simulink model "TV_2017old"  (R2016a)
settings: Solver=FixedStepAuto  StartTime=0.0  StopTime=inf  FixedStep=0.001  RelTol=1e-3
PreLoadFcn:
  | TV_2017_parameters
values from neighbouring files (symbols this model uses):
  battery_voltage = single(530)    [HIL_parameters.m]    (also in HIL_parameters_2018.m; TV_2017_parameters.m; TV_2017_parameters_VD.m)
  car_params = Simulink_Car_params    [HIL_parameters.m]    (also in HIL_parameters_2018.m; TV_2017_parameters.m; TV_2017_parameters_VD.m)
  i_Diff = 16    [HIL_parameters.m]    (also in HIL_parameters_2018.m; TV_2017_parameters.m)
  Kp = 1    [HIL_parameters.m]    (also in HIL_parameters_2018.m; TV_2017_parameters.m; TV_2017_parameters_VD.m)
  motor_data = struct    [HIL_parameters.m]    (also in HIL_parameters_2018.m; TV_2017_parameters.m)
  powerLimitControl = Simulink_el    [HIL_parameters.m]    (also in HIL_parameters_2018.m; TV_2017_parameters.m; TV_2017_parameters_VD.m)
  settings = Simulink_Settings    [HIL_parameters.m]    (also in HIL_parameters_2018.m; TV_2017_parameters.m; TV_2017_parameters_VD.m)
  SpdC_BCC = 0    [HIL_parameters.m]    (also in HIL_parameters_2018.m; TV_2017_parameters.m; TV_2017_parameters_VD.m)
  Speed_Neg_sat = -21    [HIL_parameters.m]    (also in HIL_parameters_2018.m; TV_2017_parameters.m; TV_2017_parameters_VD.m)
  Speed_Pos_sat = 21    [HIL_parameters.m]    (also in HIL_parameters_2018.m; TV_2017_parameters.m; TV_2017_parameters_VD.m)
  SteeringAngleFL = [-23.80 -22.65 -21.50 -20.34 -19.18 -18.03 -16.86 -15.70 -14.53 -13.35 -12.18 -10.99 -9.80 -8.61 -7.40 -6.19 -4.97 -3.75 -2.51 -1.26 0 1.27 2.56 3.85 5.17 6.50 7.84 9.21 10.59 12.00 13.42 14.88 16.36 17.87 19.41 20.99 22.61 24.26 25.97 27.73 29.54]    [CarSetupAnalysis2018.m]    (also in HIL_parameters_2018.m; TV_2017_parameters.m; TV_2017_parameters_VD.m = [-24.129 -22.950 -21.772 -20.593 -19.413 -18.232 -17.050 -15)
  SteeringAngleFR = [-29.54 -27.73 -25.97 -24.26 -22.61 -20.99 -19.41 -17.87 -16.36 -14.88 -13.42 -12.00 -10.59 -9.21 -7.84 -6.50 -5.17 -3.85 -2.56 -1.27 0 1.26 2.51 3.75 4.97 6.19 7.40 8.61 9.80 10.99 12.18 13.35 14.53 15.70 16.86 18.03 19.18 20.34 21.50 22.65 23.80]    [CarSetupAnalysis2018.m]    (also in HIL_parameters_2018.m; TV_2017_parameters.m; TV_2017_parameters_VD.m = [-29.3050 -27.5340 -25.8140 -24.1410 -22.5110 -20.9180 -19.3)
  SteeringWhAngle = [-105 -99.75 -94.5 -89.25 -84 -78.75 -73.5 -68.25 -63 -57.75 -52.5 -47.25 -42 -36.75 -31.5 -26.25 -21.0 -15.75 -10.5 -5.25 0.0 5.25 10.50 15.75 21.00 26.25 31.50 36.75 42.00 47.25 52.50 57.75  63.00 68.25 73.50 78.75 84.00 89.25 94.50 99.75 105.00]    [TV_2017_parameters_VD.m]
  Tn_n = 0    [HIL_parameters.m]    (also in HIL_parameters_2018.m; TV_2017_parameters.m; TV_2017_parameters_VD.m)
  tractionControl = Simulink_tc    [HIL_parameters.m]    (also in HIL_parameters_2018.m; IterativeTractionControlTuning.m; TV_2017_parameters.m; TV_2017_parameters_VD.m)
  yawRateControl = Simulink_yawRate    [HIL_parameters.m]    (also in HIL_parameters_2018.m; TV_2017_parameters.m; TV_2017_parameters_VD.m)
undefined symbols (not defined in the file or in its folder): DiscIntNeverNeededParam, magnitude, speedEstimation, TC_Decr_Gas, TC_Derivative, TC_Incr_Gas, TC_On, TC_Relay_Off, TC_Relay_On
libraries: CarMaker4SL x274, simulink_extras x45, simulink x37, dspfdesign x2
(part 4 of 14)

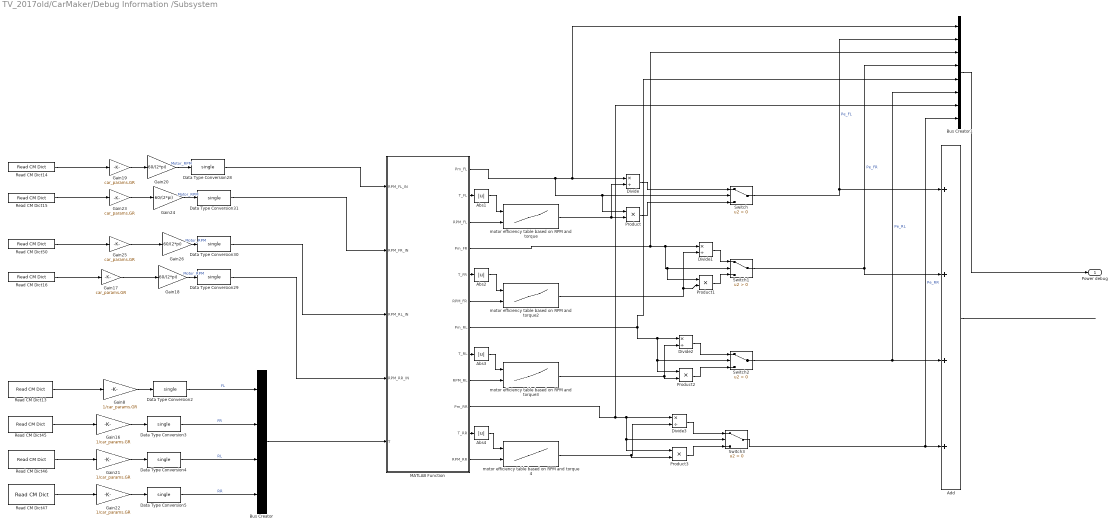
== system TV_2017old/CarMaker/Debug Information /Subsystem ==
  Abs{1..4} (4 alike) : Abs
  Add : Sum  Inputs=++++
  Bus Creator : BusCreator  Inputs=4  OutDataTypeStr=Bus: T_meas
      settings: InheritFromInputs=off
  Bus Creator1 : BusCreator  Inputs=8  OutDataTypeStr=Bus: PowerDebug
      settings: InheritFromInputs=off
  Data Type Conversion{2..5,28..31} (8 alike) : DataTypeConversion  OutDataTypeStr=single
  Divide{,1..3} (4 alike) : Product  Inputs=*/
  Gain{8,16,21..22} (4 alike) : Gain  Gain=1/car_params.GR
  Gain{17,19,23,25} (4 alike) : Gain  Gain=car_params.GR
  Gain{18,20,24,26} (4 alike) : Gain  Gain=60/(2*pi)
  MATLAB Function : MATLAB Function  TreatAsAtomicUnit=on
  Product{,1..3} (4 alike) : Product
  Read CM Dict13 : CarMaker4SL/Read CM Dict  xname=PT.WFL.Trq_Drive  xsync=off
  Read CM Dict14 : CarMaker4SL/Read CM Dict  xname=Car.WheelSpd_FL  xsync=off
  Read CM Dict15 : CarMaker4SL/Read CM Dict  xname=Car.WheelSpd_FR  xsync=off
  Read CM Dict16 : CarMaker4SL/Read CM Dict  xname=Car.WheelSpd_RR  xsync=off
  Read CM Dict45 : CarMaker4SL/Read CM Dict  xname=PT.WFR.Trq_Drive  xsync=off
  Read CM Dict46 : CarMaker4SL/Read CM Dict  xname=PT.WRL.Trq_Drive  xsync=off
  Read CM Dict47 : CarMaker4SL/Read CM Dict  xname=PT.WRR.Trq_Drive  xsync=off
  Read CM Dict50 : CarMaker4SL/Read CM Dict  xname=Car.WheelSpd_RL  xsync=off
  Switch{,1..3} (4 alike) : Switch  Criteria=u2 > Threshold
  motor efficiency table based on RPM and torque : Lookup_n-D  BreakpointsForDimension1=single([1.3,2.7,5.4,7.9,10.4,12.5,14.4,16.0,17.4,18.5,19.6]);  BreakpointsForDimension2=single([500,1000,2000,3000,4000,6000,10000,12000,15000,19000]);  Table=single(reshape([0.6437000036239624,0.5799999833106995,0.44999998807907104,0.3499999940395355,0.28999999165534973,0.23999999463558197,0.20000000298023224,0.17000000178813934,0.14000000059604645,0.12999999523162842,0.10999999940395355,0.7099999785423279,0.699999988079071,0.6100000143051148,0.5099999904632568,0.4399999976158142,0.3799999952316284,0.33000001311302185,0.28999999165534973,0.25,0.2199999988079071,0.20000000298023224,0.7300000190734863,0.7699999809265137,0.7300000190734863,0.6700000166893005,0.6100000143051148,0.550000011920929,0.5,0.44999998807907104,0.4000000059604645,0.36000001430511475,0.33000001311302185,0.7400000095367432,0.800000011920929,0.7900000214576721,0.7400000095367432,0.6899999976158142,0.6399999856948853,0.5899999737739563,0.5400000214576721,0.5,0.46000000834465027,0.41999998688697815,0.75,0.8199999928474426,0.8199999928474426,0.7799999713897705,0.7400000095367432,0.699999988079071,0.6600000262260437,0.6100000143051148,0.5699999928474426,0.5299999713897705,0.49000000953674316,0.7599999904632568,0.8399999737739563,0.8500000238418579,0.8299999833106995,0.800000011920929,0.7699999809265137,0.7400000095367432,0.699999988079071,0.6600000262260437,0.6200000047683716,0.5899999737739563,0.7699999809265137,0.8500000238418579,0.8799999952316284,0.8700000047683716,0.8600000143051148,0.8399999737739563,0.8100000023841858,0.7799999713897705,0.7599999904632568,0.7200000286102295,0.699999988079071,0.7699999809265137,0.8500000238418579,0.8899999856948853,0.8799999952316284,0.8700000047683716,0.8500000238418579,0.8299999833106995,0.8100000023841858,0.7799999713897705,0.7599999904632568,0.7300000190734863,0.7699999809265137,0.8600000143051148,0.8999999761581421,0.8999999761581421,0.8899999856948853,0.8700000047683716,0.8500000238418579,0.8299999833106995,0.8100000023841858,0.7900000214576721,0.6700000166893005,0.7799999713897705,0.8600000143051148,0.8999999761581421,0.9100000262260437,0.8999999761581421,0.8899999856948853,0.8700000047683716,0.8600000143051148,0.8299999833106995,0.7699999809265137,0.699999988079071],11,10));  ExtrapMethod=Clip  UseLastTableValue=on  InternalRulePriority=Speed  RndMeth=Simplest  InputSameDT=on
  motor efficiency table based on RPM and torque 4 : Lookup_n-D  BreakpointsForDimension1=single([1.3,2.7,5.4,7.9,10.4,12.5,14.4,16.0,17.4,18.5,19.6]);  BreakpointsForDimension2=single([500,1000,2000,3000,4000,6000,10000,12000,15000,19000]);  Table=single(reshape([0.6437000036239624,0.5799999833106995,0.44999998807907104,0.3499999940395355,0.28999999165534973,0.23999999463558197,0.20000000298023224,0.17000000178813934,0.14000000059604645,0.12999999523162842,0.10999999940395355,0.7099999785423279,0.699999988079071,0.6100000143051148,0.5099999904632568,0.4399999976158142,0.3799999952316284,0.33000001311302185,0.28999999165534973,0.25,0.2199999988079071,0.20000000298023224,0.7300000190734863,0.7699999809265137,0.7300000190734863,0.6700000166893005,0.6100000143051148,0.550000011920929,0.5,0.44999998807907104,0.4000000059604645,0.36000001430511475,0.33000001311302185,0.7400000095367432,0.800000011920929,0.7900000214576721,0.7400000095367432,0.6899999976158142,0.6399999856948853,0.5899999737739563,0.5400000214576721,0.5,0.46000000834465027,0.41999998688697815,0.75,0.8199999928474426,0.8199999928474426,0.7799999713897705,0.7400000095367432,0.699999988079071,0.6600000262260437,0.6100000143051148,0.5699999928474426,0.5299999713897705,0.49000000953674316,0.7599999904632568,0.8399999737739563,0.8500000238418579,0.8299999833106995,0.800000011920929,0.7699999809265137,0.7400000095367432,0.699999988079071,0.6600000262260437,0.6200000047683716,0.5899999737739563,0.7699999809265137,0.8500000238418579,0.8799999952316284,0.8700000047683716,0.8600000143051148,0.8399999737739563,0.8100000023841858,0.7799999713897705,0.7599999904632568,0.7200000286102295,0.699999988079071,0.7699999809265137,0.8500000238418579,0.8899999856948853,0.8799999952316284,0.8700000047683716,0.8500000238418579,0.8299999833106995,0.8100000023841858,0.7799999713897705,0.7599999904632568,0.7300000190734863,0.7699999809265137,0.8600000143051148,0.8999999761581421,0.8999999761581421,0.8899999856948853,0.8700000047683716,0.8500000238418579,0.8299999833106995,0.8100000023841858,0.7900000214576721,0.6700000166893005,0.7799999713897705,0.8600000143051148,0.8999999761581421,0.9100000262260437,0.8999999761581421,0.8899999856948853,0.8700000047683716,0.8600000143051148,0.8299999833106995,0.7699999809265137,0.699999988079071],11,10));  ExtrapMethod=Clip  UseLastTableValue=on  InternalRulePriority=Speed  RndMeth=Simplest  InputSameDT=on
  motor efficiency table based on RPM and torque2 : Lookup_n-D  BreakpointsForDimension1=single([1.3,2.7,5.4,7.9,10.4,12.5,14.4,16.0,17.4,18.5,19.6]);  BreakpointsForDimension2=single([500,1000,2000,3000,4000,6000,10000,12000,15000,19000]);  Table=single(reshape([0.6437000036239624,0.5799999833106995,0.44999998807907104,0.3499999940395355,0.28999999165534973,0.23999999463558197,0.20000000298023224,0.17000000178813934,0.14000000059604645,0.12999999523162842,0.10999999940395355,0.7099999785423279,0.699999988079071,0.6100000143051148,0.5099999904632568,0.4399999976158142,0.3799999952316284,0.33000001311302185,0.28999999165534973,0.25,0.2199999988079071,0.20000000298023224,0.7300000190734863,0.7699999809265137,0.7300000190734863,0.6700000166893005,0.6100000143051148,0.550000011920929,0.5,0.44999998807907104,0.4000000059604645,0.36000001430511475,0.33000001311302185,0.7400000095367432,0.800000011920929,0.7900000214576721,0.7400000095367432,0.6899999976158142,0.6399999856948853,0.5899999737739563,0.5400000214576721,0.5,0.46000000834465027,0.41999998688697815,0.75,0.8199999928474426,0.8199999928474426,0.7799999713897705,0.7400000095367432,0.699999988079071,0.6600000262260437,0.6100000143051148,0.5699999928474426,0.5299999713897705,0.49000000953674316,0.7599999904632568,0.8399999737739563,0.8500000238418579,0.8299999833106995,0.800000011920929,0.7699999809265137,0.7400000095367432,0.699999988079071,0.6600000262260437,0.6200000047683716,0.5899999737739563,0.7699999809265137,0.8500000238418579,0.8799999952316284,0.8700000047683716,0.8600000143051148,0.8399999737739563,0.8100000023841858,0.7799999713897705,0.7599999904632568,0.7200000286102295,0.699999988079071,0.7699999809265137,0.8500000238418579,0.8899999856948853,0.8799999952316284,0.8700000047683716,0.8500000238418579,0.8299999833106995,0.8100000023841858,0.7799999713897705,0.7599999904632568,0.7300000190734863,0.7699999809265137,0.8600000143051148,0.8999999761581421,0.8999999761581421,0.8899999856948853,0.8700000047683716,0.8500000238418579,0.8299999833106995,0.8100000023841858,0.7900000214576721,0.6700000166893005,0.7799999713897705,0.8600000143051148,0.8999999761581421,0.9100000262260437,0.8999999761581421,0.8899999856948853,0.8700000047683716,0.8600000143051148,0.8299999833106995,0.7699999809265137,0.699999988079071],11,10));  ExtrapMethod=Clip  UseLastTableValue=on  InternalRulePriority=Speed  RndMeth=Simplest  InputSameDT=on
  motor efficiency table based on RPM and torque3 : Lookup_n-D  BreakpointsForDimension1=single([1.3,2.7,5.4,7.9,10.4,12.5,14.4,16.0,17.4,18.5,19.6]);  BreakpointsForDimension2=single([500,1000,2000,3000,4000,6000,10000,12000,15000,19000]);  Table=single(reshape([0.6437000036239624,0.5799999833106995,0.44999998807907104,0.3499999940395355,0.28999999165534973,0.23999999463558197,0.20000000298023224,0.17000000178813934,0.14000000059604645,0.12999999523162842,0.10999999940395355,0.7099999785423279,0.699999988079071,0.6100000143051148,0.5099999904632568,0.4399999976158142,0.3799999952316284,0.33000001311302185,0.28999999165534973,0.25,0.2199999988079071,0.20000000298023224,0.7300000190734863,0.7699999809265137,0.7300000190734863,0.6700000166893005,0.6100000143051148,0.550000011920929,0.5,0.44999998807907104,0.4000000059604645,0.36000001430511475,0.33000001311302185,0.7400000095367432,0.800000011920929,0.7900000214576721,0.7400000095367432,0.6899999976158142,0.6399999856948853,0.5899999737739563,0.5400000214576721,0.5,0.46000000834465027,0.41999998688697815,0.75,0.8199999928474426,0.8199999928474426,0.7799999713897705,0.7400000095367432,0.699999988079071,0.6600000262260437,0.6100000143051148,0.5699999928474426,0.5299999713897705,0.49000000953674316,0.7599999904632568,0.8399999737739563,0.8500000238418579,0.8299999833106995,0.800000011920929,0.7699999809265137,0.7400000095367432,0.699999988079071,0.6600000262260437,0.6200000047683716,0.5899999737739563,0.7699999809265137,0.8500000238418579,0.8799999952316284,0.8700000047683716,0.8600000143051148,0.8399999737739563,0.8100000023841858,0.7799999713897705,0.7599999904632568,0.7200000286102295,0.699999988079071,0.7699999809265137,0.8500000238418579,0.8899999856948853,0.8799999952316284,0.8700000047683716,0.8500000238418579,0.8299999833106995,0.8100000023841858,0.7799999713897705,0.7599999904632568,0.7300000190734863,0.7699999809265137,0.8600000143051148,0.8999999761581421,0.8999999761581421,0.8899999856948853,0.8700000047683716,0.8500000238418579,0.8299999833106995,0.8100000023841858,0.7900000214576721,0.6700000166893005,0.7799999713897705,0.8600000143051148,0.8999999761581421,0.9100000262260437,0.8999999761581421,0.8899999856948853,0.8700000047683716,0.8600000143051148,0.8299999833106995,0.7699999809265137,0.699999988079071],11,10));  ExtrapMethod=Clip  UseLastTableValue=on  InternalRulePriority=Speed  RndMeth=Simplest  InputSameDT=on
  Power debug : Outport
  wires:
  motor efficiency table based on RPM and torque 4/1 -> Product3/2, Divide3/2
  motor efficiency table based on RPM and torque3/1 -> Product2/2, Divide2/2
  Divide1/1 -> Switch1/1
  Product1/1 -> Switch1/3
  MATLAB Function/3(RPM_FL) -> motor efficiency table based on RPM and torque/2
  MATLAB Function/10(Pm_RR) -> Bus Creator1/7, Switch3/2, Product3/1, Divide3/1
  MATLAB Function/2(T_FL) -> Abs1/1
  MATLAB Function/8(T_RL) -> Abs3/1
  Abs4/1 -> motor efficiency table based on RPM and torque 4/1
  Abs2/1 -> motor efficiency table based on RPM and torque2/1
  Data Type Conversion28/1 -> MATLAB Function/1(RPM_FL_IN)
  MATLAB Function/5(T_FR) -> Abs2/1
  MATLAB Function/11(T_RR) -> Abs4/1
  MATLAB Function/12(RPM_RR) -> motor efficiency table based on RPM and torque 4/2
  MATLAB Function/1(Pm_FL) -> Product/1, Switch/2, Divide/1, Bus Creator1/1
  MATLAB Function/7(Pm_RL) -> Switch2/2, Product2/1, Divide2/1, Bus Creator1/5
  Data Type Conversion31/1 -> MATLAB Function/2(RPM_FR_IN)
  Data Type Conversion30/1 -> MATLAB Function/3(RPM_RL_IN)
  Divide/1 -> Switch/1
  Product/1 -> Switch/3
  Data Type Conversion29/1 -> MATLAB Function/4(RPM_RR_IN)
  Bus Creator/1 -> MATLAB Function/5(T)
  motor efficiency table based on RPM and torque/1 -> Divide/2, Product/2
  MATLAB Function/4(Pm_FR) -> Bus Creator1/3, Product1/1, Switch1/2, Divide1/1
  Abs1/1 -> motor efficiency table based on RPM and torque/1
  motor efficiency table based on RPM and torque2/1 -> Divide1/2, Product1/2
  MATLAB Function/6(RPM_FR) -> motor efficiency table based on RPM and torque2/2
  Switch/1 -> Bus Creator1/2, Add/1  "Pe_FL"
  MATLAB Function/9(RPM_RL) -> motor efficiency table based on RPM and torque3/2
  Abs3/1 -> motor efficiency table based on RPM and torque3/1
  Divide2/1 -> Switch2/1
  Divide3/1 -> Switch3/1
  Read CM Dict13/1 -> Gain8/1
  Read CM Dict46/1 -> Gain21/1
  Read CM Dict45/1 -> Gain16/1
  Product3/1 -> Switch3/3
  Switch2/1 -> Bus Creator1/6, Add/3  "Pe_RL"
  Product2/1 -> Switch2/3
  Switch1/1 -> Bus Creator1/4, Add/2  "Pe_FR"
  Switch3/1 -> Add/4, Bus Creator1/8  "Pe_RR"
  Gain24/1 -> Data Type Conversion31/1  "Motor_RPM"
  Read CM Dict15/1 -> Gain23/1
  Gain8/1 -> Data Type Conversion2/1
  Gain22/1 -> Data Type Conversion5/1
  Read CM Dict50/1 -> Gain25/1
  Gain23/1 -> Gain24/1
  Gain19/1 -> Gain20/1
  Bus Creator1/1 -> Power debug/1
  Gain18/1 -> Data Type Conversion29/1  "Motor_RPM"
  Gain26/1 -> Data Type Conversion30/1  "Motor_RPM"
  Read CM Dict14/1 -> Gain19/1
  Data Type Conversion4/1 -> Bus Creator/3  "RL"
  Add/1 -> ?
  Read CM Dict16/1 -> Gain17/1
  Gain17/1 -> Gain18/1
  Data Type Conversion3/1 -> Bus Creator/2  "FR"
  Gain25/1 -> Gain26/1
  Gain16/1 -> Data Type Conversion3/1
  Gain21/1 -> Data Type Conversion4/1
  Data Type Conversion2/1 -> Bus Creator/1  "FL"
  Gain20/1 -> Data Type Conversion28/1  "Motor_RPM"
  Data Type Conversion5/1 -> Bus Creator/4  "RR"
  Read CM Dict47/1 -> Gain22/1

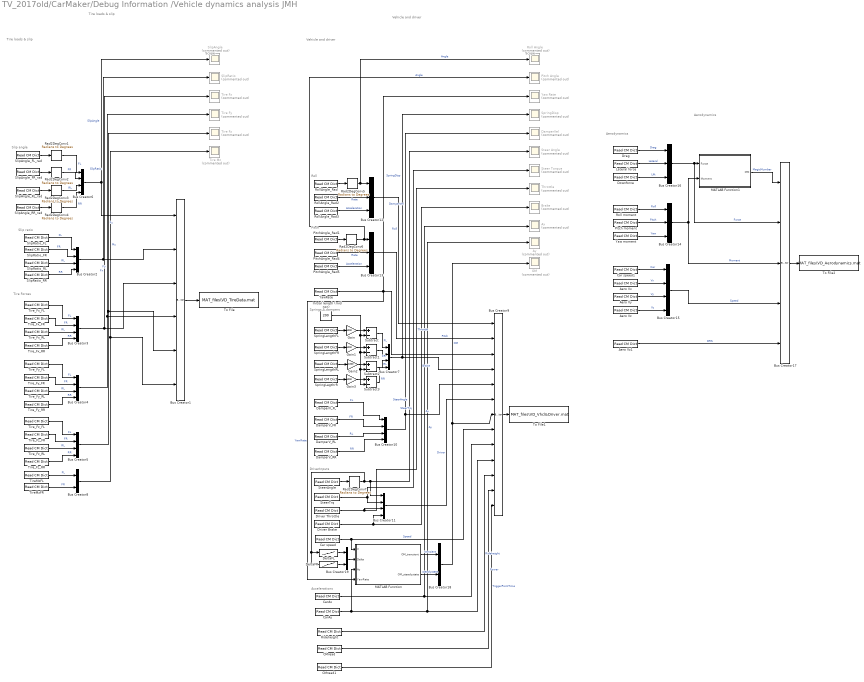
== system TV_2017old/CarMaker/Debug Information /Vehicle dynamics analysis JMH ==
  note: Aerodynamics
  note: Vehicle and driver
  note: Tire loads & slip
  note: Aerodynamics
  note: Tire loads & slip
  note: Vehicle and driver
  note: Tire Forces
  note: Scope
  note: Slip ratio
  note: Slip angle
  note: Scope
  note: Springs & dampers
  note: DriverInputs
  note: Roll
  note: Pitch
  note: Accelerations
  Aero Vx : CarMaker4SL/Read CM Dict  xname=Car.Aero.vres_1.x  xsync=off
  Aero Vy : CarMaker4SL/Read CM Dict  xname=Car.Aero.vres_1.y  xsync=off
  Aero Vz : CarMaker4SL/Read CM Dict  xname=Car.Aero.vres_1.z  xsync=off
  Aero Vz1 : CarMaker4SL/Read CM Dict  xname=DRS  xsync=off
  Ax : Scope  Commented=on
  Ay : Scope  Commented=on
  Brake : Scope  Commented=on
  Bus Creator1 : BusCreator  Inputs=6
  Bus Creator{2..7,10..11,15} (9 alike) : BusCreator  Inputs=4
  Bus Creator{12..14,16} (4 alike) : BusCreator  Inputs=3
  Bus Creator17 : BusCreator  Inputs=5
  Bus Creator18 : BusCreator  Inputs=2
  Bus Creator19 : BusCreator  Inputs=2
  Bus Creator8 : BusCreator  Inputs=2
  Bus Creator9 : BusCreator  Inputs=13
  CMread : CarMaker4SL/Read CM Dict  xname=Power  xsync=off
  CMread1 : CarMaker4SL/Read CM Dict  xname=DM.TriggerPoint.Time  xsync=off
  Car speed : CarMaker4SL/Read CM Dict  xname=Vhcl.v  xsync=off
  Car speed1 : CarMaker4SL/Read CM Dict  xname=Vhcl.v  xsync=off
  CarAx : CarMaker4SL/Read CM Dict  xname=Car.ax  xsync=off
  CarAy : CarMaker4SL/Read CM Dict  xname=Car.ay  xsync=off
  DamperV_FL : CarMaker4SL/Read CM Dict  xname=Car.DampFL.v  xsync=off
  DamperV_FR : CarMaker4SL/Read CM Dict  xname=Car.SpringFR.l  xsync=off
  DamperV_RL : CarMaker4SL/Read CM Dict  xname=Car.SpringRL.l  xsync=off
  DamperV_RR : CarMaker4SL/Read CM Dict  xname=Car.SpringRR.l  xsync=off
  DamperVel : Scope  Commented=on
  DeltaFL : Lookup_n-D  NumberOfTableDimensions=1  BreakpointsForDimension1=SteeringWhAngle  Table=SteeringAngleFL  InterpMethod=Cubic spline  ExtrapMethod=Clip  InternalRulePriority=Speed  RndMeth=Simplest  InputSameDT=on
  DeltaFR : Lookup_n-D  NumberOfTableDimensions=1  BreakpointsForDimension1=SteeringWhAngle  Table=SteeringAngleFR  InterpMethod=Cubic spline  ExtrapMethod=Clip  InternalRulePriority=Speed  RndMeth=Simplest  InputSameDT=on
  Downforce : CarMaker4SL/Read CM Dict  xname=Car.Aero.Frc_1.z  xsync=off
  Drag : CarMaker4SL/Read CM Dict  xname=Car.Aero.Frc_1.x  xsync=off
  Driver Brake : CarMaker4SL/Read CM Dict  xname=DM.Brake  xsync=off
  "Driver Throttle " : CarMaker4SL/Read CM Dict  xname=DM.Gas  xsync=off
  Gain{,1..3} (4 alike) : Gain  Gain=1000
  Initial length (mid pos) : Constant  Value=200
  Lateral force : CarMaker4SL/Read CM Dict  xname=Car.Aero.Frc_1.y  xsync=off
  MATLAB Function : MATLAB Function  TreatAsAtomicUnit=on
  MATLAB Function1 : MATLAB Function  TreatAsAtomicUnit=on
  OM : Scope  Commented=on
  Pitch Angle : Scope  Commented=on
  Pitch moment : CarMaker4SL/Read CM Dict  xname=Car.Aero.Trq_1.y  xsync=off
  PitchAngle_Rad1 : CarMaker4SL/Read CM Dict  xname=Vhcl.Pitch  xsync=off
  PitchAngle_Rad4 : CarMaker4SL/Read CM Dict  xname=Vhcl.PitchVel  xsync=off
  PitchAngle_Rad5 : CarMaker4SL/Read CM Dict  xname=Vhcl.PitchAcc  xsync=off
  Rad2DegConv{1..7} (7 alike) : simulink_extras/Transformations/Radians to Degrees
  Rideheight : CarMaker4SL/Read CM Dict  xname=RideHeight  xsync=off
  Roll Angle : Scope  Commented=on
  Roll moment : CarMaker4SL/Read CM Dict  xname=Car.Aero.Trq_1.x  xsync=off
  RollAngle_Rad : CarMaker4SL/Read CM Dict  xname=Vhcl.Roll  xsync=off
  RollAngle_Rad2 : CarMaker4SL/Read CM Dict  xname=Vhcl.RollVel  xsync=off
  RollAngle_Rad3 : CarMaker4SL/Read CM Dict  xname=Vhcl.RollAcc  xsync=off
  SlipAngle : Scope  Commented=on
  SlipAngle_FL_rad : CarMaker4SL/Read CM Dict  xname=Car.SlipAngleFL  xsync=off
  SlipAngle_FR_rad : CarMaker4SL/Read CM Dict  xname=Car.SlipAngleFR  xsync=off
  SlipAngle_RL_rad : CarMaker4SL/Read CM Dict  xname=Car.SlipAngleRL  xsync=off
  SlipAngle_RR_rad : CarMaker4SL/Read CM Dict  xname=Car.SlipAngleRR  xsync=off
  SlipRatio : Scope  Commented=on
  SlipRatio_FL : CarMaker4SL/Read CM Dict  xname=Car.LongSlipFL  xsync=off
  SlipRatio_FR : CarMaker4SL/Read CM Dict  xname=Car.LongSlipFR  xsync=off
  SlipRatio_RL : CarMaker4SL/Read CM Dict  xname=Car.LongSlipRL  xsync=off
  SlipRatio_RR : CarMaker4SL/Read CM Dict  xname=Car.LongSlipRR  xsync=off
  SpringDisp : Scope  Commented=on
  SpringLegthrR : CarMaker4SL/Read CM Dict  xname=Car.SpringRR.l  xsync=off
  SpringLengthFL : CarMaker4SL/Read CM Dict  xname=Car.SpringFL.l  xsync=off
  SpringLengthFR : CarMaker4SL/Read CM Dict  xname=Car.SpringFR.l  xsync=off
  SpringLengthRL : CarMaker4SL/Read CM Dict  xname=Car.SpringRL.l  xsync=off
  Steer Angle : Scope  Commented=on
  Steer Torque : Scope  Commented=on
  SteerAngle : CarMaker4SL/Read CM Dict  xname=DM.Steer.Ang  xsync=off
  SteerTrq : CarMaker4SL/Read CM Dict  xname=DM.Steer.Trq  xsync=off
  Subtract{,1..3} (4 alike) : Sum  Inputs=+-
  Throttle : Scope  Commented=on
  Tire Fx : Scope  Commented=on
  Tire Fy : Scope  Commented=on
  Tire Fz : Scope  Commented=on
  Tire Mz : Scope  Commented=on
  TireMzFL : CarMaker4SL/Read CM Dict  xname=Car.TrqAlignFL  xsync=off
  TireMzFR : CarMaker4SL/Read CM Dict  xname=Car.TrqAlignFR  xsync=off
  Tire_Fx_FL : CarMaker4SL/Read CM Dict  xname=Car.FxFL  xsync=off
  Tire_Fx_FR : CarMaker4SL/Read CM Dict  xname=Car.FxFR  xsync=off
  Tire_Fx_RL : CarMaker4SL/Read CM Dict  xname=Car.FxRL  xsync=off
  Tire_Fx_RR : CarMaker4SL/Read CM Dict  xname=Car.FxRR  xsync=off
  Tire_Fy_FL : CarMaker4SL/Read CM Dict  xname=Car.FyFL  xsync=off
  Tire_Fy_FR : CarMaker4SL/Read CM Dict  xname=Car.FyFR  xsync=off
  Tire_Fy_RL : CarMaker4SL/Read CM Dict  xname=Car.FyRL  xsync=off
  Tire_Fy_RR : CarMaker4SL/Read CM Dict  xname=Car.FyRR  xsync=off
  Tire_Fz_FL : CarMaker4SL/Read CM Dict  xname=Car.FzFL  xsync=off
  Tire_Fz_FR : CarMaker4SL/Read CM Dict  xname=Car.FzFR  xsync=off
  Tire_Fz_RL : CarMaker4SL/Read CM Dict  xname=Car.FzRL  xsync=off
  Tire_Fz_RR : CarMaker4SL/Read CM Dict  xname=Car.FzRR  xsync=off
  To File : ToFile  Filename=MAT_files\VD_TireData.mat  MatrixName=Tire  SaveFormat=Timeseries
  To File1 : ToFile  Filename=MAT_files\VD_Vhcl&Driver.mat  MatrixName=Vhcl  SaveFormat=Timeseries
  To File2 : ToFile  Filename=MAT_files\VD_Aerodynamics.mat  MatrixName=Aero  SaveFormat=Timeseries
  Yaw Rate : Scope  Commented=on
  Yaw moment : CarMaker4SL/Read CM Dict  xname=Car.Aero.Trq_1.z  xsync=off
  YawRate : CarMaker4SL/Read CM Dict  xname=Car.YawRate  xsync=off
  wires:
  TireMzFR/1 -> Bus Creator8/2  "FR"
  TireMzFL/1 -> Bus Creator8/1  "FL"
  Bus Creator8/1 -> Bus Creator1/6, Tire Mz/1  "Mz"
  Tire_Fx_RR/1 -> Bus Creator3/4  "RR"
  Tire_Fx_RL/1 -> Bus Creator3/3  "RL"
  Rad2DegConv1/1 -> Bus Creator6/1  "FL"
  Rad2DegConv2/1 -> Bus Creator6/2  "FR"
  Bus Creator1/1 -> To File/1
  SlipAngle_RR_rad/1 -> Rad2DegConv4/1
  Tire_Fx_FL/1 -> Bus Creator3/1  "FL"
  Tire_Fy_FR/1 -> Bus Creator4/2  "FR"
  Bus Creator4/1 -> Tire Fy/1, Bus Creator1/4  "Fy"
  Bus Creator5/1 -> Bus Creator1/5, Tire Fz/1  "Fz"
  SlipAngle_RL_rad/1 -> Rad2DegConv3/1
  Tire_Fz_RL/1 -> Bus Creator5/3  "RL"
  Tire_Fz_FL/1 -> Bus Creator5/1  "FL"
  SlipRatio_RL/1 -> Bus Creator2/3  "RL"
  Tire_Fz_FR/1 -> Bus Creator5/2  "FR"
  Tire_Fy_RL/1 -> Bus Creator4/3  "RL"
  Tire_Fy_RR/1 -> Bus Creator4/4  "RR"
  SlipRatio_FR/1 -> Bus Creator2/2  "FR"
  Bus Creator2/1 -> Bus Creator1/2, SlipRatio/1  "SlipRatio"
  SlipAngle_FL_rad/1 -> Rad2DegConv1/1
  Rad2DegConv4/1 -> Bus Creator6/4  "RR"
  SlipAngle_FR_rad/1 -> Rad2DegConv2/1
  Rad2DegConv3/1 -> Bus Creator6/3  "RL"
  Tire_Fz_RR/1 -> Bus Creator5/4  "RR"
  SlipRatio_FL/1 -> Bus Creator2/1  "FL"
  Bus Creator6/1 -> SlipAngle/1, Bus Creator1/1  "SlipAngle"
  SlipRatio_RR/1 -> Bus Creator2/4  "RR"
  Tire_Fx_FR/1 -> Bus Creator3/2  "FR"
  Tire_Fy_FL/1 -> Bus Creator4/1  "FL"
  Bus Creator3/1 -> Bus Creator1/3, Tire Fx/1  "Fx"
  Car speed/1 -> MATLAB Function/1(V), Bus Creator9/8  "Speed"
  MATLAB Function/1(OM_transient) -> Bus Creator18/1  "transient"
  Bus Creator13/1 -> Bus Creator9/2  "Pitch"
  PitchAngle_Rad5/1 -> Bus Creator13/3  "Acceleration"
  PitchAngle_Rad4/1 -> Bus Creator13/2  "Rate"
  RollAngle_Rad3/1 -> Bus Creator12/3  "Acceleration"
  Bus Creator12/1 -> Bus Creator9/1  "Roll"
  RollAngle_Rad2/1 -> Bus Creator12/2  "Rate"
  Subtract3/1 -> Bus Creator7/4  "RR"
  Gain2/1 -> Subtract2/1
  Subtract2/1 -> Bus Creator7/3  "RL"
  Gain1/1 -> Subtract1/1
  Gain/1 -> Subtract/1
  "Driver Throttle "/1 -> Throttle/1, Bus Creator11/3  "Throttle"
  Bus Creator11/1 -> Bus Creator9/6  "Driver"
  Subtract/1 -> Bus Creator7/1  "FL"
  Initial length (mid pos)/1 -> Subtract1/2, Subtract2/2, Subtract3/2, Subtract/2
  RollAngle_Rad/1 -> Rad2DegConv5/1
  Bus Creator7/1 -> Bus Creator9/4, SpringDisp/1  "SpringDisp"
  SpringLengthFL/1 -> Gain/1
  SpringLengthFR/1 -> Gain1/1
  Rad2DegConv5/1 -> Roll Angle/1, Bus Creator12/1  "Angle"
  PitchAngle_Rad1/1 -> Rad2DegConv6/1
  Rad2DegConv6/1 -> Pitch Angle/1, Bus Creator13/1  "Angle"
  SpringLengthRL/1 -> Gain2/1
  Bus Creator9/1 -> To File1/1
  SpringLegthrR/1 -> Gain3/1
  YawRate/1 -> Yaw Rate/1, Bus Creator9/3, MATLAB Function/4(YawRate)  "YawRate"
  DamperV_FR/1 -> Bus Creator10/2  "FR"
  Rad2DegConv7/1 -> DeltaFL/1, DeltaFR/1, Steer Angle/1, Bus Creator11/1  "SteerAngle"
  Driver Brake/1 -> Brake/1, Bus Creator11/4  "Brake"
  SteerTrq/1 -> Steer Torque/1, Bus Creator11/2  "SteerTrq"
  SteerAngle/1 -> Rad2DegConv7/1
  DamperV_FL/1 -> Bus Creator10/1  "FL"
  DamperV_RR/1 -> Bus Creator10/4  "RR"
  DamperV_RL/1 -> Bus Creator10/3  "RL"
  Bus Creator10/1 -> Bus Creator9/5, DamperVel/1  "DamperVel"
  Subtract1/1 -> Bus Creator7/2  "FR"
  Gain3/1 -> Subtract3/1
  Car speed1/1 -> Bus Creator15/1  "Car"
  Bus Creator15/1 -> Bus Creator17/4  "Speed"
  Aero Vz/1 -> Bus Creator15/4  "Vz"
  Aero Vy/1 -> Bus Creator15/3  "Vy"
  Aero Vx/1 -> Bus Creator15/2  "Vx"
  Bus Creator14/1 -> MATLAB Function1/2(Moment), Bus Creator17/3  "Moment"
  Bus Creator16/1 -> MATLAB Function1/1(Force), Bus Creator17/2  "Force"
  MATLAB Function1/1(MM) -> Bus Creator17/1  "MagicMumber"
  Bus Creator17/1 -> To File2/1
  Yaw moment/1 -> Bus Creator14/3  "Yaw"
  Pitch moment/1 -> Bus Creator14/2  "Pitch"
  Roll moment/1 -> Bus Creator14/1  "Roll"
  Downforce/1 -> Bus Creator16/3  "Lift"
  Lateral force/1 -> Bus Creator16/2  "Lateral"
  Drag/1 -> Bus Creator16/1  "Drag"
  CarAx/1 -> Bus Creator9/9, Ax/1  "Ax"
  CarAy/1 -> MATLAB Function/3(Ay), Bus Creator9/10, Ay/1  "Ay"
  MATLAB Function/2(OM_steadystate) -> Bus Creator18/2  "steadystate"
  Bus Creator18/1 -> OM/1, Bus Creator9/7  "OM"
  DeltaFR/1 -> Bus Creator19/2
  DeltaFL/1 -> Bus Creator19/1
  Bus Creator19/1 -> MATLAB Function/2(Delta)
  Aero Vz1/1 -> Bus Creator17/5  "DRS"
  Rideheight/1 -> Bus Creator9/11  "Rideheight"
  CMread/1 -> Bus Creator9/12  "Power"
  CMread1/1 -> Bus Creator9/13  "TriggerPointTime"

== system TV_2017old/CarMaker/Debug Information /add_elements ==
  In1 : Inport
  Demux : Demux
  Sum1 : Sum  Inputs=|++
  Sum2 : Sum  Inputs=|++
  Sum3 : Sum  Inputs=|++
  Out1 : Outport
  wires:
  In1/1 -> Demux/1
  Demux/3 -> Sum3/1
  Demux/4 -> Sum3/2
  Sum3/1 -> Sum2/2
  Sum2/1 -> Sum1/2
  Demux/2 -> Sum2/1
  Demux/1 -> Sum1/1
  Sum1/1 -> Out1/1

== system TV_2017old/CarMaker/Debug Information /addall ==
  In1 : Inport
  Demux : Demux
  Sum : Sum  Inputs=|++
  Sum1 : Sum  Inputs=|++
  Sum2 : Sum  Inputs=|++
  Out1 : Outport
  wires:
  Sum2/1 -> Out1/1
  Demux/1 -> Sum/1
  Sum/1 -> Sum1/1
  Sum1/1 -> Sum2/1
  Demux/2 -> Sum/2
  Demux/3 -> Sum1/2
  Demux/4 -> Sum2/2
  In1/1 -> Demux/1

== system TV_2017old/CarMaker/Debug Information /addall1 ==
  In1 : Inport
  Demux : Demux
  Sum : Sum  Inputs=|++
  Sum1 : Sum  Inputs=|++
  Sum2 : Sum  Inputs=|++
  Out1 : Outport
  wires:
  Sum2/1 -> Out1/1
  Demux/1 -> Sum/1
  Sum/1 -> Sum1/1
  Sum1/1 -> Sum2/1
  Demux/2 -> Sum/2
  Demux/3 -> Sum1/2
  Demux/4 -> Sum2/2
  In1/1 -> Demux/1

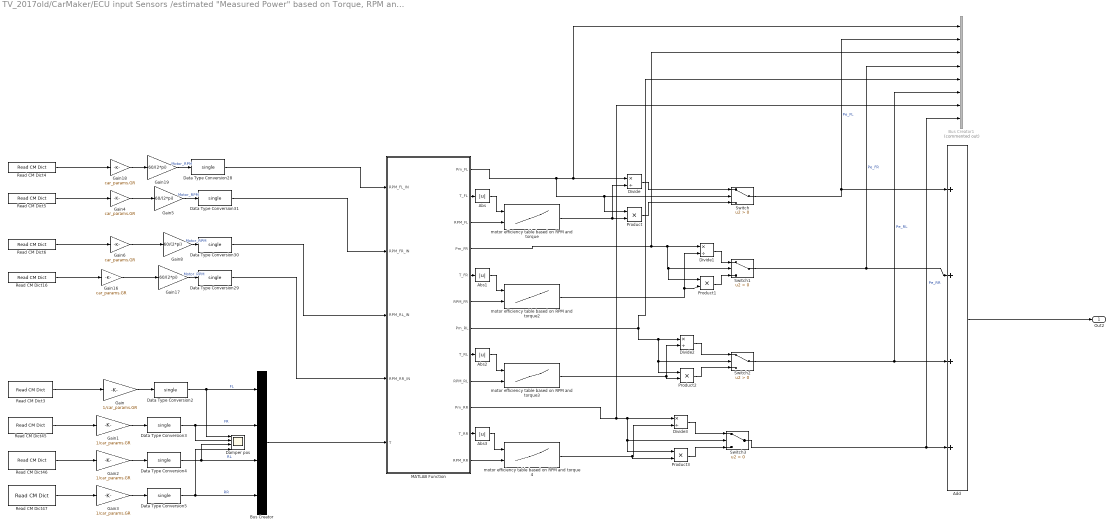
== system TV_2017old/CarMaker/ECU input Sensors /estimated "Measured Power" based on Torque, RPM and datasheet IRL this is measured ==
  Abs{,1..3} (4 alike) : Abs
  Add : Sum  Inputs=++++
  Bus Creator : BusCreator  Inputs=4  OutDataTypeStr=Bus: T_meas
      settings: InheritFromInputs=off
  Bus Creator1 : BusCreator  Commented=on  Inputs=8  OutDataTypeStr=Bus: PowerDebug
      settings: InheritFromInputs=off
  Damper pos : Scope  NumInputPorts=4
  Data Type Conversion{2..5,28..31} (8 alike) : DataTypeConversion  OutDataTypeStr=single
  Divide{,1..3} (4 alike) : Product  Inputs=*/
  Gain{,1..3} (4 alike) : Gain  Gain=1/car_params.GR
  Gain{4,6,16,18} (4 alike) : Gain  Gain=car_params.GR
  Gain{5,8,17,19} (4 alike) : Gain  Gain=60/(2*pi)
  MATLAB Function : MATLAB Function  TreatAsAtomicUnit=on
  Product{,1..3} (4 alike) : Product
  Read CM Dict16 : CarMaker4SL/Read CM Dict  xname=Car.WheelSpd_RR  xsync=off
  Read CM Dict3 : CarMaker4SL/Read CM Dict  xname=PT.WFL.Trq_Drive  xsync=off
  Read CM Dict4 : CarMaker4SL/Read CM Dict  xname=Car.WheelSpd_FL  xsync=off
  Read CM Dict45 : CarMaker4SL/Read CM Dict  xname=PT.WFR.Trq_Drive  xsync=off
  Read CM Dict46 : CarMaker4SL/Read CM Dict  xname=PT.WRL.Trq_Drive  xsync=off
  Read CM Dict47 : CarMaker4SL/Read CM Dict  xname=PT.WRR.Trq_Drive  xsync=off
  Read CM Dict5 : CarMaker4SL/Read CM Dict  xname=Car.WheelSpd_FR  xsync=off
  Read CM Dict6 : CarMaker4SL/Read CM Dict  xname=Car.WheelSpd_RL  xsync=off
  Switch{,1..3} (4 alike) : Switch  Criteria=u2 > Threshold
  motor efficiency table based on RPM and torque : Lookup_n-D  BreakpointsForDimension1=single([1.3,2.7,5.4,7.9,10.4,12.5,14.4,16.0,17.4,18.5,19.6]);  BreakpointsForDimension2=single([500,1000,2000,3000,4000,6000,10000,12000,15000,19000]);  Table=single(reshape([0.6437000036239624,0.5799999833106995,0.44999998807907104,0.3499999940395355,0.28999999165534973,0.23999999463558197,0.20000000298023224,0.17000000178813934,0.14000000059604645,0.12999999523162842,0.10999999940395355,0.7099999785423279,0.699999988079071,0.6100000143051148,0.5099999904632568,0.4399999976158142,0.3799999952316284,0.33000001311302185,0.28999999165534973,0.25,0.2199999988079071,0.20000000298023224,0.7300000190734863,0.7699999809265137,0.7300000190734863,0.6700000166893005,0.6100000143051148,0.550000011920929,0.5,0.44999998807907104,0.4000000059604645,0.36000001430511475,0.33000001311302185,0.7400000095367432,0.800000011920929,0.7900000214576721,0.7400000095367432,0.6899999976158142,0.6399999856948853,0.5899999737739563,0.5400000214576721,0.5,0.46000000834465027,0.41999998688697815,0.75,0.8199999928474426,0.8199999928474426,0.7799999713897705,0.7400000095367432,0.699999988079071,0.6600000262260437,0.6100000143051148,0.5699999928474426,0.5299999713897705,0.49000000953674316,0.7599999904632568,0.8399999737739563,0.8500000238418579,0.8299999833106995,0.800000011920929,0.7699999809265137,0.7400000095367432,0.699999988079071,0.6600000262260437,0.6200000047683716,0.5899999737739563,0.7699999809265137,0.8500000238418579,0.8799999952316284,0.8700000047683716,0.8600000143051148,0.8399999737739563,0.8100000023841858,0.7799999713897705,0.7599999904632568,0.7200000286102295,0.699999988079071,0.7699999809265137,0.8500000238418579,0.8899999856948853,0.8799999952316284,0.8700000047683716,0.8500000238418579,0.8299999833106995,0.8100000023841858,0.7799999713897705,0.7599999904632568,0.7300000190734863,0.7699999809265137,0.8600000143051148,0.8999999761581421,0.8999999761581421,0.8899999856948853,0.8700000047683716,0.8500000238418579,0.8299999833106995,0.8100000023841858,0.7900000214576721,0.6700000166893005,0.7799999713897705,0.8600000143051148,0.8999999761581421,0.9100000262260437,0.8999999761581421,0.8899999856948853,0.8700000047683716,0.8600000143051148,0.8299999833106995,0.7699999809265137,0.699999988079071],11,10));  ExtrapMethod=Clip  UseLastTableValue=on  InternalRulePriority=Speed  RndMeth=Simplest  InputSameDT=on
  motor efficiency table based on RPM and torque 4 : Lookup_n-D  BreakpointsForDimension1=single([1.3,2.7,5.4,7.9,10.4,12.5,14.4,16.0,17.4,18.5,19.6]);  BreakpointsForDimension2=single([500,1000,2000,3000,4000,6000,10000,12000,15000,19000]);  Table=single(reshape([0.6437000036239624,0.5799999833106995,0.44999998807907104,0.3499999940395355,0.28999999165534973,0.23999999463558197,0.20000000298023224,0.17000000178813934,0.14000000059604645,0.12999999523162842,0.10999999940395355,0.7099999785423279,0.699999988079071,0.6100000143051148,0.5099999904632568,0.4399999976158142,0.3799999952316284,0.33000001311302185,0.28999999165534973,0.25,0.2199999988079071,0.20000000298023224,0.7300000190734863,0.7699999809265137,0.7300000190734863,0.6700000166893005,0.6100000143051148,0.550000011920929,0.5,0.44999998807907104,0.4000000059604645,0.36000001430511475,0.33000001311302185,0.7400000095367432,0.800000011920929,0.7900000214576721,0.7400000095367432,0.6899999976158142,0.6399999856948853,0.5899999737739563,0.5400000214576721,0.5,0.46000000834465027,0.41999998688697815,0.75,0.8199999928474426,0.8199999928474426,0.7799999713897705,0.7400000095367432,0.699999988079071,0.6600000262260437,0.6100000143051148,0.5699999928474426,0.5299999713897705,0.49000000953674316,0.7599999904632568,0.8399999737739563,0.8500000238418579,0.8299999833106995,0.800000011920929,0.7699999809265137,0.7400000095367432,0.699999988079071,0.6600000262260437,0.6200000047683716,0.5899999737739563,0.7699999809265137,0.8500000238418579,0.8799999952316284,0.8700000047683716,0.8600000143051148,0.8399999737739563,0.8100000023841858,0.7799999713897705,0.7599999904632568,0.7200000286102295,0.699999988079071,0.7699999809265137,0.8500000238418579,0.8899999856948853,0.8799999952316284,0.8700000047683716,0.8500000238418579,0.8299999833106995,0.8100000023841858,0.7799999713897705,0.7599999904632568,0.7300000190734863,0.7699999809265137,0.8600000143051148,0.8999999761581421,0.8999999761581421,0.8899999856948853,0.8700000047683716,0.8500000238418579,0.8299999833106995,0.8100000023841858,0.7900000214576721,0.6700000166893005,0.7799999713897705,0.8600000143051148,0.8999999761581421,0.9100000262260437,0.8999999761581421,0.8899999856948853,0.8700000047683716,0.8600000143051148,0.8299999833106995,0.7699999809265137,0.699999988079071],11,10));  ExtrapMethod=Clip  UseLastTableValue=on  InternalRulePriority=Speed  RndMeth=Simplest  InputSameDT=on
  motor efficiency table based on RPM and torque2 : Lookup_n-D  BreakpointsForDimension1=single([1.3,2.7,5.4,7.9,10.4,12.5,14.4,16.0,17.4,18.5,19.6]);  BreakpointsForDimension2=single([500,1000,2000,3000,4000,6000,10000,12000,15000,19000]);  Table=single(reshape([0.6437000036239624,0.5799999833106995,0.44999998807907104,0.3499999940395355,0.28999999165534973,0.23999999463558197,0.20000000298023224,0.17000000178813934,0.14000000059604645,0.12999999523162842,0.10999999940395355,0.7099999785423279,0.699999988079071,0.6100000143051148,0.5099999904632568,0.4399999976158142,0.3799999952316284,0.33000001311302185,0.28999999165534973,0.25,0.2199999988079071,0.20000000298023224,0.7300000190734863,0.7699999809265137,0.7300000190734863,0.6700000166893005,0.6100000143051148,0.550000011920929,0.5,0.44999998807907104,0.4000000059604645,0.36000001430511475,0.33000001311302185,0.7400000095367432,0.800000011920929,0.7900000214576721,0.7400000095367432,0.6899999976158142,0.6399999856948853,0.5899999737739563,0.5400000214576721,0.5,0.46000000834465027,0.41999998688697815,0.75,0.8199999928474426,0.8199999928474426,0.7799999713897705,0.7400000095367432,0.699999988079071,0.6600000262260437,0.6100000143051148,0.5699999928474426,0.5299999713897705,0.49000000953674316,0.7599999904632568,0.8399999737739563,0.8500000238418579,0.8299999833106995,0.800000011920929,0.7699999809265137,0.7400000095367432,0.699999988079071,0.6600000262260437,0.6200000047683716,0.5899999737739563,0.7699999809265137,0.8500000238418579,0.8799999952316284,0.8700000047683716,0.8600000143051148,0.8399999737739563,0.8100000023841858,0.7799999713897705,0.7599999904632568,0.7200000286102295,0.699999988079071,0.7699999809265137,0.8500000238418579,0.8899999856948853,0.8799999952316284,0.8700000047683716,0.8500000238418579,0.8299999833106995,0.8100000023841858,0.7799999713897705,0.7599999904632568,0.7300000190734863,0.7699999809265137,0.8600000143051148,0.8999999761581421,0.8999999761581421,0.8899999856948853,0.8700000047683716,0.8500000238418579,0.8299999833106995,0.8100000023841858,0.7900000214576721,0.6700000166893005,0.7799999713897705,0.8600000143051148,0.8999999761581421,0.9100000262260437,0.8999999761581421,0.8899999856948853,0.8700000047683716,0.8600000143051148,0.8299999833106995,0.7699999809265137,0.699999988079071],11,10));  ExtrapMethod=Clip  UseLastTableValue=on  InternalRulePriority=Speed  RndMeth=Simplest  InputSameDT=on
  motor efficiency table based on RPM and torque3 : Lookup_n-D  BreakpointsForDimension1=single([1.3,2.7,5.4,7.9,10.4,12.5,14.4,16.0,17.4,18.5,19.6]);  BreakpointsForDimension2=single([500,1000,2000,3000,4000,6000,10000,12000,15000,19000]);  Table=single(reshape([0.6437000036239624,0.5799999833106995,0.44999998807907104,0.3499999940395355,0.28999999165534973,0.23999999463558197,0.20000000298023224,0.17000000178813934,0.14000000059604645,0.12999999523162842,0.10999999940395355,0.7099999785423279,0.699999988079071,0.6100000143051148,0.5099999904632568,0.4399999976158142,0.3799999952316284,0.33000001311302185,0.28999999165534973,0.25,0.2199999988079071,0.20000000298023224,0.7300000190734863,0.7699999809265137,0.7300000190734863,0.6700000166893005,0.6100000143051148,0.550000011920929,0.5,0.44999998807907104,0.4000000059604645,0.36000001430511475,0.33000001311302185,0.7400000095367432,0.800000011920929,0.7900000214576721,0.7400000095367432,0.6899999976158142,0.6399999856948853,0.5899999737739563,0.5400000214576721,0.5,0.46000000834465027,0.41999998688697815,0.75,0.8199999928474426,0.8199999928474426,0.7799999713897705,0.7400000095367432,0.699999988079071,0.6600000262260437,0.6100000143051148,0.5699999928474426,0.5299999713897705,0.49000000953674316,0.7599999904632568,0.8399999737739563,0.8500000238418579,0.8299999833106995,0.800000011920929,0.7699999809265137,0.7400000095367432,0.699999988079071,0.6600000262260437,0.6200000047683716,0.5899999737739563,0.7699999809265137,0.8500000238418579,0.8799999952316284,0.8700000047683716,0.8600000143051148,0.8399999737739563,0.8100000023841858,0.7799999713897705,0.7599999904632568,0.7200000286102295,0.699999988079071,0.7699999809265137,0.8500000238418579,0.8899999856948853,0.8799999952316284,0.8700000047683716,0.8500000238418579,0.8299999833106995,0.8100000023841858,0.7799999713897705,0.7599999904632568,0.7300000190734863,0.7699999809265137,0.8600000143051148,0.8999999761581421,0.8999999761581421,0.8899999856948853,0.8700000047683716,0.8500000238418579,0.8299999833106995,0.8100000023841858,0.7900000214576721,0.6700000166893005,0.7799999713897705,0.8600000143051148,0.8999999761581421,0.9100000262260437,0.8999999761581421,0.8899999856948853,0.8700000047683716,0.8600000143051148,0.8299999833106995,0.7699999809265137,0.699999988079071],11,10));  ExtrapMethod=Clip  UseLastTableValue=on  InternalRulePriority=Speed  RndMeth=Simplest  InputSameDT=on
  Out2 : Outport
  wires:
  MATLAB Function/3(RPM_FL) -> motor efficiency table based on RPM and torque/2
  Data Type Conversion28/1 -> MATLAB Function/1(RPM_FL_IN)
  MATLAB Function/2(T_FL) -> Abs/1
  motor efficiency table based on RPM and torque 4/1 -> Product3/2, Divide3/2
  Divide1/1 -> Switch1/1
  Product1/1 -> Switch1/3
  MATLAB Function/10(Pm_RR) -> Bus Creator1/7, Switch3/2, Product3/1, Divide3/1
  motor efficiency table based on RPM and torque3/1 -> Product2/2, Divide2/2
  MATLAB Function/8(T_RL) -> Abs2/1
  Abs3/1 -> motor efficiency table based on RPM and torque 4/1
  Abs1/1 -> motor efficiency table based on RPM and torque2/1
  Bus Creator/1 -> MATLAB Function/5(T)
  MATLAB Function/12(RPM_RR) -> motor efficiency table based on RPM and torque 4/2
  MATLAB Function/1(Pm_FL) -> Product/1, Switch/2, Divide/1, Bus Creator1/1
  MATLAB Function/7(Pm_RL) -> Switch2/2, Product2/1, Divide2/1, Bus Creator1/5
  MATLAB Function/5(T_FR) -> Abs1/1
  MATLAB Function/11(T_RR) -> Abs3/1
  Data Type Conversion31/1 -> MATLAB Function/2(RPM_FR_IN)
  MATLAB Function/9(RPM_RL) -> motor efficiency table based on RPM and torque3/2
  Data Type Conversion30/1 -> MATLAB Function/3(RPM_RL_IN)
  Data Type Conversion29/1 -> MATLAB Function/4(RPM_RR_IN)
  Divide/1 -> Switch/1
  Product/1 -> Switch/3
  Abs2/1 -> motor efficiency table based on RPM and torque3/1
  motor efficiency table based on RPM and torque/1 -> Divide/2, Product/2
  MATLAB Function/4(Pm_FR) -> Bus Creator1/3, Product1/1, Switch1/2, Divide1/1
  Abs/1 -> motor efficiency table based on RPM and torque/1
  motor efficiency table based on RPM and torque2/1 -> Divide1/2, Product1/2
  MATLAB Function/6(RPM_FR) -> motor efficiency table based on RPM and torque2/2
  Switch/1 -> Bus Creator1/2, Add/1  "Pe_FL"
  Divide2/1 -> Switch2/1
  Product3/1 -> Switch3/3
  Switch2/1 -> Bus Creator1/6, Add/3  "Pe_RL"
  Product2/1 -> Switch2/3
  Switch1/1 -> Bus Creator1/4, Add/2  "Pe_FR"
  Switch3/1 -> Add/4, Bus Creator1/8  "Pe_RR"
  Divide3/1 -> Switch3/1
  Read CM Dict46/1 -> Gain2/1
  Read CM Dict3/1 -> Gain/1
  Read CM Dict45/1 -> Gain1/1
  Gain6/1 -> Gain8/1
  Data Type Conversion2/1 -> Damper pos/1, Bus Creator/1  "FL"
  Gain2/1 -> Data Type Conversion4/1
  Read CM Dict4/1 -> Gain18/1
  Read CM Dict6/1 -> Gain6/1
  Gain17/1 -> Data Type Conversion29/1  "Motor_RPM"
  Data Type Conversion5/1 -> Damper pos/4, Bus Creator/4  "RR"
  Gain/1 -> Data Type Conversion2/1
  Gain3/1 -> Data Type Conversion5/1
  Gain4/1 -> Gain5/1
  Read CM Dict47/1 -> Gain3/1
  Gain1/1 -> Data Type Conversion3/1
  Gain5/1 -> Data Type Conversion31/1  "Motor_RPM"
  Gain8/1 -> Data Type Conversion30/1  "Motor_RPM"
  Data Type Conversion4/1 -> Damper pos/3, Bus Creator/3  "RL"
  Data Type Conversion3/1 -> Damper pos/2, Bus Creator/2  "FR"
  Gain18/1 -> Gain19/1
  Read CM Dict16/1 -> Gain16/1
  Add/1 -> Out2/1
  Read CM Dict5/1 -> Gain4/1
  Gain16/1 -> Gain17/1
  Gain19/1 -> Data Type Conversion28/1  "Motor_RPM"

== system TV_2017old/CarMaker/Estimations/1st_deriv ==
  signal : Inport
  Diff_Function : MATLAB Function  TreatAsAtomicUnit=on
  Memory : Memory  X0=[0;0;0;0;0;0;0;0;0;0;0;0;0;0;0]  InheritSampleTime=on
  delta_t : Constant  Value=0.01
  deriv : Outport
  deriv1 : Outport  Port=2
  wires:
  delta_t/1 -> Diff_Function/3(delta_t)
  Diff_Function/2(y) -> deriv/1
  signal/1 -> Diff_Function/2(sensors)
  Diff_Function/1(y_old) -> Memory/1
  Memory/1 -> Diff_Function/1("y_old ")
  Diff_Function/3(RPM_der) -> deriv1/1

== system TV_2017old/CarMaker/Estimations/EstimateVx ==
  sensors : Inport
  Fz_est : Inport  Port=2
  velocity_Estimation : MATLAB Function  TreatAsAtomicUnit=on
  v_x_est : Outport
  wires:
  sensors/1 -> velocity_Estimation/1(sensors)
  Fz_est/1 -> velocity_Estimation/2(normalForces)
  velocity_Estimation/1(V_est_x) -> v_x_est/1

== system TV_2017old/CarMaker/Estimations/Fx_Estimation ==
  sensors : Inport
  EstimateFx : MATLAB Function  TreatAsAtomicUnit=on
  T_motor : Outport
  Fx : Outport  Port=2
  wires:
  sensors/1 -> EstimateFx/1(sensors)
  EstimateFx/1(Fx) -> Fx/1
  EstimateFx/2(T_motor) -> T_motor/1

== system TV_2017old/CarMaker/Estimations/Fz_Estimation ==
  sensors : Inport
  1st_deriv : Subsystem
  2nd_deriv : Subsystem
  Bus Selector : BusSelector  OutputSignals=damper_rate_FL,damper_rate_FR,damper_rate_RL,damper_rate_RR
  Bus Selector1 : BusSelector  OutputSignals=FL,FR,RL,RR
  DamperRateLookup : Lookup_n-D  NumberOfTableDimensions=1  BreakpointsForDimension1=car_params.damper_table_breakpoint;  Table=car_params.damper_pull_push_values_front;  ExtrapMethod=Clip  UseLastTableValue=on  InternalRulePriority=Speed  RndMeth=Simplest  InputSameDT=on
  DamperRateLookup1 : Lookup_n-D  NumberOfTableDimensions=1  BreakpointsForDimension1=car_params.damper_table_breakpoint;  Table=car_params.damper_pull_push_values_front;  ExtrapMethod=Clip  UseLastTableValue=on  InternalRulePriority=Speed  RndMeth=Simplest  InputSameDT=on
  DamperRateLookup2 : Lookup_n-D  NumberOfTableDimensions=1  BreakpointsForDimension1=car_params.damper_table_breakpoint;  Table=car_params.damper_pull_push_values_rear;  ExtrapMethod=Clip  UseLastTableValue=on  InternalRulePriority=Speed  RndMeth=Simplest  InputSameDT=on
  DamperRateLookup3 : Lookup_n-D  NumberOfTableDimensions=1  BreakpointsForDimension1=car_params.damper_table_breakpoint;  Table=car_params.damper_pull_push_values_rear;  ExtrapMethod=Clip  UseLastTableValue=on  InternalRulePriority=Speed  RndMeth=Simplest  InputSameDT=on
  FZ_etsimate : Scope  NumInputPorts=4
  FzEstDamper : MATLAB Function  TreatAsAtomicUnit=on
  Scope2 : Scope  NumInputPorts=4
  Sum : Sum  Inputs=|++++
  Sum_FZ : Scope
  alfa_r_scope : Scope
  Fz_est : Outport
  Fz_damper_est : Outport  Port=2
  alfa_r : Outport  Port=3
  wires:
  sensors/1 -> FzEstDamper/1(sensors), Bus Selector/1
  Bus Selector/1 -> DamperRateLookup/1  "<damper_rate_FL>"
  Bus Selector/2 -> DamperRateLookup1/1  "<damper_rate_FR>"
  Bus Selector/3 -> DamperRateLookup2/1  "<damper_rate_RL>"
  Bus Selector/4 -> DamperRateLookup3/1  "<damper_rate_RR>"
  FzEstDamper/2(alfa_r) -> alfa_r_scope/1, alfa_r/1
  Bus Selector1/2 -> Sum/3, FZ_etsimate/2  "<FR>"
  Bus Selector1/1 -> Sum/4, FZ_etsimate/1  "<FL>"
  Bus Selector1/3 -> Sum/2, FZ_etsimate/3  "<RL>"
  Bus Selector1/4 -> FZ_etsimate/4, Sum/1  "<RR>"
  FzEstDamper/1(Fz_damper_est) -> Bus Selector1/1, Fz_est/1, Fz_damper_est/1
  DamperRateLookup1/1 -> Scope2/2, FzEstDamper/3(Fz_damp_FR)  "<FR>"
  DamperRateLookup/1 -> Scope2/1, FzEstDamper/2(Fz_damp_FL)  "<FL>"
  DamperRateLookup2/1 -> Scope2/3, FzEstDamper/4(Fz_damp_RL)  "<RL>"
  DamperRateLookup3/1 -> Scope2/4, FzEstDamper/5(Fz_damp_RR)  "<RR>"
  Sum/1 -> Sum_FZ/1

== system TV_2017old/CarMaker/Estimations/Fz_Estimation_acceleration based ==
  sensors : Inport
  Bus Selector1 : BusSelector  OutputSignals=FL,FR,RL,RR
  Bus Selector2 : BusSelector  OutputSignals=Input_throttle,Input_brake,KERS_pos
  FZ_etsimate_acceleration : Scope  NumInputPorts=4
  Fz_acc_est : MATLAB Function  TreatAsAtomicUnit=on
  LowPassFilter : Subsystem
  Lowpass Filter : dspfdesign/Lowpass Filter  FilterType=FIR  DesignForMinimumOrder=on  FilterOrder=50  PassbandFrequency=4  StopbandFrequency=15  PassbandRipple=0.1  StopbandAttenuation=80  InheritSampleRate=on  SampleRate=100  roundingMode=Floor  coeffsDataTypeStr=fixdt(1,16)  SimulateUsing=Interpreted execution
  Lowpass Filter1 : dspfdesign/Lowpass Filter  FilterType=FIR  DesignForMinimumOrder=on  FilterOrder=50  PassbandFrequency=4  StopbandFrequency=15  PassbandRipple=0.1  StopbandAttenuation=80  InheritSampleRate=on  SampleRate=100  roundingMode=Floor  coeffsDataTypeStr=fixdt(1,16)  SimulateUsing=Code generation
  alfa_r_acc : Scope  NumInputPorts=2
  alfa_r_acc_tps_bps_kers : Scope  NumInputPorts=4
  filtervsUnfilter : Scope  NumInputPorts=2
  Out1 : Outport
  wires:
  sensors/1 -> Bus Selector2/1, Fz_acc_est/1(sensors)
  Bus Selector1/2 -> FZ_etsimate_acceleration/2  "<FR>"
  Bus Selector1/1 -> Lowpass Filter/1, LowPassFilter/1(In1), filtervsUnfilter/2, FZ_etsimate_acceleration/1  "<FL>"
  Bus Selector1/3 -> FZ_etsimate_acceleration/3  "<RL>"
  Bus Selector1/4 -> FZ_etsimate_acceleration/4  "<RR>"
  Fz_acc_est/1(Fz_acc_est) -> Out1/1, Bus Selector1/1
  Lowpass Filter/1 -> filtervsUnfilter/1
  Lowpass Filter1/1 -> alfa_r_acc/1
  Fz_acc_est/2(alfa_r_acc) -> alfa_r_acc_tps_bps_kers/1, alfa_r_acc/2, Lowpass Filter1/1
  Bus Selector2/1 -> alfa_r_acc_tps_bps_kers/2  "<Input_throttle>"
  Bus Selector2/2 -> alfa_r_acc_tps_bps_kers/3  "<Input_brake>"
  Bus Selector2/3 -> alfa_r_acc_tps_bps_kers/4  "<KERS_pos>"

== system TV_2017old/CarMaker/Estimations/RPM_to_linearVelocity ==
  sensors : Inport
  meanWheelAngle : Inport  Port=2
  whl_v_calculation : MATLAB Function  TreatAsAtomicUnit=on
  whl_speed : Outport
  wires:
  whl_v_calculation/1(whl_speed) -> whl_speed/1
  sensors/1 -> whl_v_calculation/1(sensors)
  meanWheelAngle/1 -> whl_v_calculation/2(meanWheelAngle)
